simulink model "testSampleModel"  (R2023b)
settings: Solver=VariableStepAuto  StartTime=0.0  StopTime=10.0  RelTol=1e-3
undefined symbols (not defined in the file or in its folder): testBusWithExample
libraries: simulink x1
settings Model: Creator=peterc  LastModifiedBy=peterc

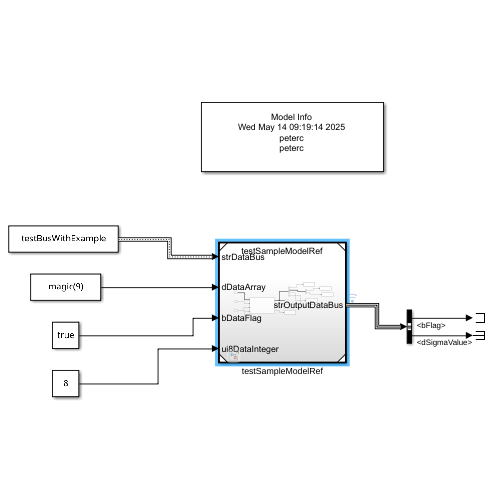
[thumbnail: Simulink's stored preview of the top-level diagram]
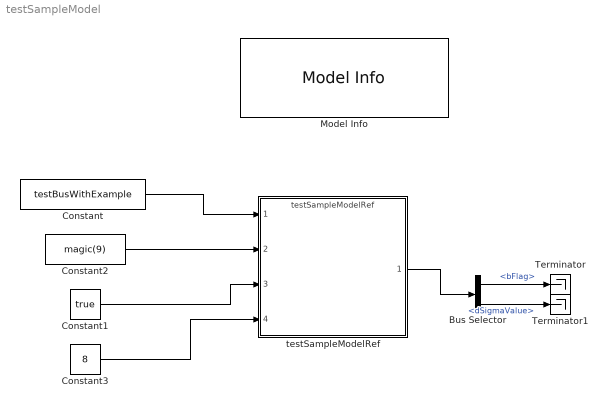
== system testSampleModel ==
  Bus Selector : BusSelector  OutputSignals=bFlag,dSigmaValue
  Constant : Constant  Value=testBusWithExample  VectorParams1D=off  OutDataTypeStr=Bus: bus_testBusWithExample
  Constant1 : Constant  Value=true  OutDataTypeStr=boolean
  Constant2 : Constant  Value=magic(9)  OutDataTypeStr=double
  Constant3 : Constant  Value=8  OutDataTypeStr=uint8
  Model Info : simulink/Model-Wide Utilities/Model Info  Frame=on  DisplayStringWithTags=|  HorizontalTextAlignment=Center  LeftAlignmentValue=0.5
      | Model Info
      | %<Created>
      | %<Creator>
      | %<ModifiedBy>
      | %<Description>
  Terminator : Terminator
  Terminator1 : Terminator
  testSampleModelRef : ModelReference  ModelNameDialog=testSampleModelRef.slx  SimulationMode=Normal  ModelReferenceVersion=1.6
  wires:
  Constant/1 -> testSampleModelRef/1
  Constant2/1 -> testSampleModelRef/2
  Constant1/1 -> testSampleModelRef/3
  Constant3/1 -> testSampleModelRef/4
  testSampleModelRef/1 -> Bus Selector/1
  Bus Selector/1 -> Terminator/1  "<bFlag>"
  Bus Selector/2 -> Terminator1/1  "<dSigmaValue>"
